simulink model "TPM_SWC"  (R2022b)
settings: configuration reference "TPS_AutosarConfig" (kept outside this file)
model workspace (MATLAB code in the model file):
  | cmdLim = Simulink.Parameter;
  | cmdLim.Value = 15;
  | cmdLim.Description = 'Limit for controlling the maximum surface command angle.';
  | cmdLim.Min = 0;
  | cmdLim.Max = 90;
  | cmdLim.DocUnits = 'deg';
  | 
  | dispGain = Simulink.Parameter;
  | dispGain.Value = 0.75;
  | dispGain.Description = 'Gain applied to the displacement error.';
  | dispGain.Min = 0;
  | dispGain.Max = [];
  | dispGain.DocUnits = 'deg/sec/deg';
  | 
  | dispLim = Simulink.Parameter;
  | dispLim.Value = 30;
  | dispLim.Description = 'Limit for controlling the maximum commanded angle.';
  | dispLim.Min = 0;
  | dispLim.Max = 180;
  | dispLim.DocUnits = 'deg';
  | 
  | intGain = Simulink.Parameter;
  | intGain.Value = 0.5;
  | intGain.Description = 'Gain applied to the integral error.';
  | intGain.Min = 0;
  | intGain.Max = [];
  | intGain.DocUnits = 'deg/sec/deg/sec';
  | 
  | intLim = Simulink.Parameter;
  | intLim.Value = 5;
  | intLim.Description = 'Limit for controlling the maximum commanded angle.';
  | intLim.Min = 0;
  | intLim.Max = 90;
  | intLim.DocUnits = 'deg';
  | 
  | rateGain = Simulink.Parameter;
  | rateGain.Value = 2;
  | rateGain.Description = 'Gain applied to the rate error.';
  | rateGain.Min = 0;
  | rateGain.Max = [];
  | rateGain.DocUnits = 'deg/deg/sec';
  | 
  | rateLim = Simulink.Parameter;
  | rateLim.Value = 6;
  | rateLim.Description = 'Limit for controlling the maximum commanded angle.';
  | rateLim.Min = 0;
  | rateLim.Max = 180;
  | rateLim.DocUnits = 'deg/sec';
  | 
  | hdgGain = Simulink.Parameter;
  | hdgGain.Value = 0.015;
values from neighbouring files (symbols this model uses):
  Dem_EventStatusType : value not decoded    [TPS_DD.sldd]
libraries: autosarlibdem x5
settings Model: RequirementInfo={} %GIDa_fe9045fd_0412_4b6e_8206_617cc20e6fde  DataDictionary=TPS_DD.sldd  FPTRunName=Active  Creator=MAAM  LastModifiedBy=MAAM
settings ConfigSetRef: SourceName=TPS_AutosarConfig

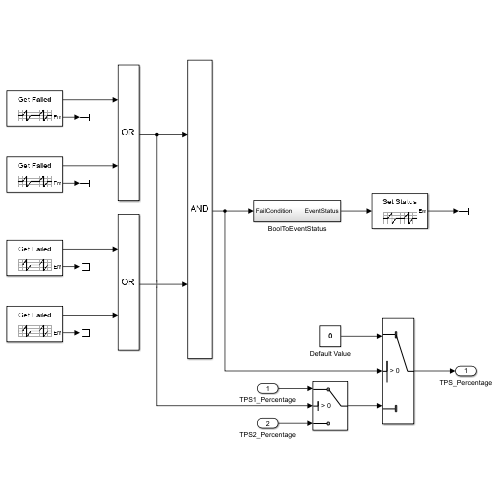
[thumbnail: Simulink's stored preview of the top-level diagram]
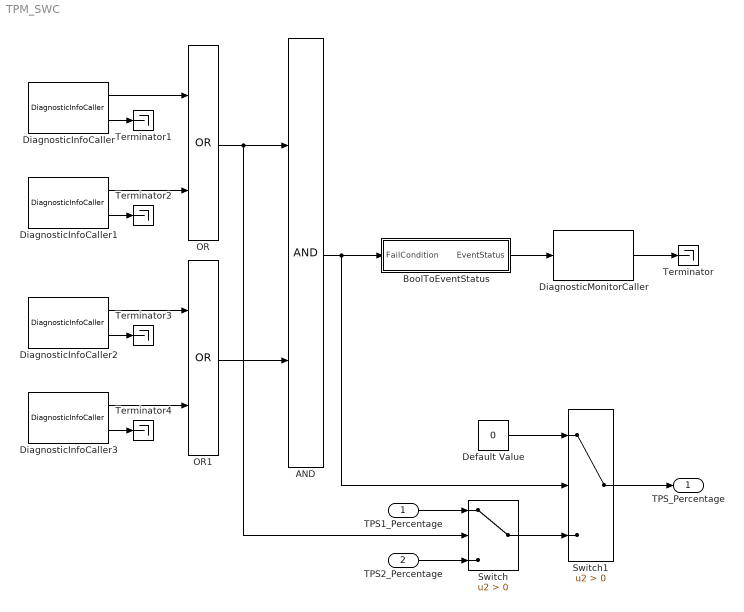
== system TPM_SWC ==
  TPS1_Percentage : Inport
  TPS2_Percentage : Inport  Port=2
  AND : Logic  AllPortsSameDT=off  OutDataTypeStr=boolean
  BoolToEventStatus : Subsystem
  Default Value : Constant  Value=0  OutDataTypeStr=single
  DiagnosticInfoCaller : autosarlibdem/DiagnosticInfoCaller  PortName=TPS1_StuckLow  Operation=GetEventFailed  st=-1  ServiceImpl=autosar.bsw.DemDiagnosticInfo
  DiagnosticInfoCaller1 : autosarlibdem/DiagnosticInfoCaller  PortName=TPS1_StuckHigh  Operation=GetEventFailed  st=-1  ServiceImpl=autosar.bsw.DemDiagnosticInfo
  DiagnosticInfoCaller2 : autosarlibdem/DiagnosticInfoCaller  PortName=TPS2_StuckLow  Operation=GetEventFailed  st=-1  ServiceImpl=autosar.bsw.DemDiagnosticInfo
  DiagnosticInfoCaller3 : autosarlibdem/DiagnosticInfoCaller  PortName=TPS2_StuckHigh  Operation=GetEventFailed  st=-1  ServiceImpl=autosar.bsw.DemDiagnosticInfo
  DiagnosticMonitorCaller : autosarlibdem/DiagnosticMonitorCaller  PortName=TPS_Fail  Operation=SetEventStatus  Datatype=Enum: Dem_EventStatusType  st=-1  ServiceImpl=autosar.bsw.DemDiagnosticMonitor
  OR : Logic  Operator=OR  AllPortsSameDT=off  OutDataTypeStr=boolean
  OR1 : Logic  Operator=OR  AllPortsSameDT=off  OutDataTypeStr=boolean
  Switch : Switch  Criteria=u2 > Threshold  SaturateOnIntegerOverflow=off  InputSameDT=off
  Switch1 : Switch  Criteria=u2 > Threshold  SaturateOnIntegerOverflow=off  InputSameDT=off
  Terminator{,1..4} (5 alike) : Terminator
  TPS_Percentage : Outport
  wires:
  TPS1_Percentage/1 -> Switch/1
  TPS2_Percentage/1 -> Switch/3
  Switch/1 -> Switch1/3
  Switch1/1 -> TPS_Percentage/1
  Default Value/1 -> Switch1/1
  DiagnosticMonitorCaller/1 -> Terminator/1
  BoolToEventStatus/1(EventStatus) -> DiagnosticMonitorCaller/1
  DiagnosticInfoCaller/2 -> Terminator1/1
  DiagnosticInfoCaller1/2 -> Terminator2/1
  DiagnosticInfoCaller2/2 -> Terminator3/1
  DiagnosticInfoCaller3/2 -> Terminator4/1
  DiagnosticInfoCaller/1 -> OR/1
  DiagnosticInfoCaller1/1 -> OR/2
  DiagnosticInfoCaller3/1 -> OR1/2
  DiagnosticInfoCaller2/1 -> OR1/1
  OR/1 -> AND/1, Switch/2
  OR1/1 -> AND/2
  AND/1 -> BoolToEventStatus/1(FailCondition), Switch1/2

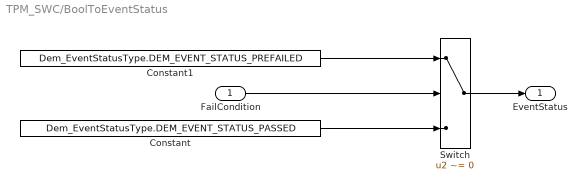
== system TPM_SWC/BoolToEventStatus ==
  FailCondition : Inport
  Constant : Constant  Value=Dem_EventStatusType.DEM_EVENT_STATUS_PASSED
  Constant1 : Constant  Value=Dem_EventStatusType.DEM_EVENT_STATUS_PREFAILED
  Switch : Switch  Criteria=u2 ~= 0  SaturateOnIntegerOverflow=off  InputSameDT=off
  EventStatus : Outport  VectorParamsAs1DForOutWhenUnconnected=off
  wires:
  FailCondition/1 -> Switch/2
  Constant/1 -> Switch/3
  Constant1/1 -> Switch/1
  Switch/1 -> EventStatus/1
